simulink model "Simulink_WMM"  (R2021a)
settings: Solver=ode1be  StartTime=0.0  StopTime=350  FixedStep=0.001  RelTol=1e-3
values from neighbouring files (symbols this model uses):
  s = cross(t,r)    [traj_plan_circle.m]
  Y = 0    [traj_plan_3priority.m]    (also in traj_plan_double2.m; traj_plan_ee_8.m; traj_plan_ee_circle.m; traj_plan_scene.m)
undefined symbols (not defined in the file or in its folder): X, Z
libraries: sm_lib x132, nesl_utility x61
(part 1 of 4)
settings Model: PacingRate=0.890000  Creator=zhouz  LastModifiedBy=zhouz

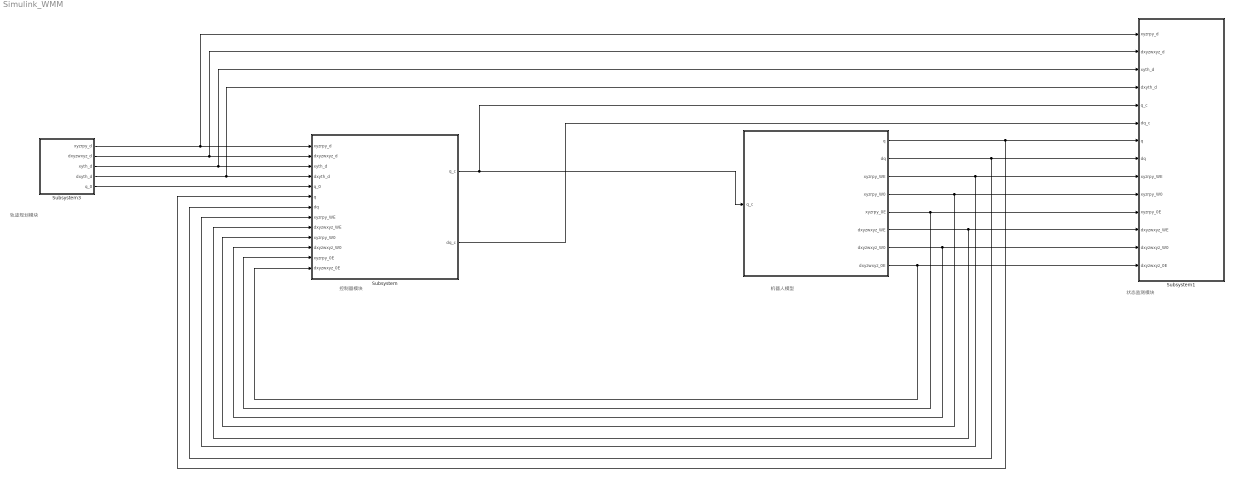
== system Simulink_WMM ==
  note: 机器人模型
  note: 状态监测模块
  note: 控制器模块
  note: 轨迹规划模块
  " " : Subsystem
  Subsystem : Subsystem
  Subsystem1 : Subsystem
  Subsystem3 : Subsystem
  wires:
  Subsystem/2(dq_c) -> Subsystem1/6(dq_c)
  Subsystem3/2(dxyzwxyz_d) -> Subsystem/2(dxyzwxyz_d), Subsystem1/2(dxyzwxyz_d)
  " "/4(xyzrpy_W0) -> Subsystem/10(xyzrpy_W0), Subsystem1/10(xyzrpy_W0)
  Subsystem3/1(xyzrpy_d) -> Subsystem1/1(xyzrpy_d), Subsystem/1(xyzrpy_d)
  Subsystem3/4(dxyth_d) -> Subsystem/4(dxyth_d), Subsystem1/4(dxyth_d)
  Subsystem3/3(xyth_d) -> Subsystem/3(xyth_d), Subsystem1/3(xyth_d)
  " "/8(dxyzwxyz_0E) -> Subsystem1/14(dxyzwxyz_0E), Subsystem/13(dxyzwxyz_0E)
  " "/5(xyzrpy_0E) -> Subsystem/12(xyzrpy_0E), Subsystem1/11(xyzrpy_0E)
  Subsystem/1(q_c) -> " "/1(q_c), Subsystem1/5(q_c)
  " "/7(dxyzwxyz_W0) -> Subsystem1/13(dxyzwxyz_W0), Subsystem/11(dxyzwxyz_W0)
  " "/6(dxyzwxyz_WE) -> Subsystem1/12(dxyzwxyz_WE), Subsystem/9(dxyzwxyz_WE)
  " "/2(dq) -> Subsystem/7(dq), Subsystem1/8(dq)
  " "/1(q) -> Subsystem/6(q), Subsystem1/7(q)
  " "/3(xyzrpy_WE) -> Subsystem/8(xyzrpy_WE), Subsystem1/9(xyzrpy_WE)
  Subsystem3/5(q_0) -> Subsystem/5(q_0)

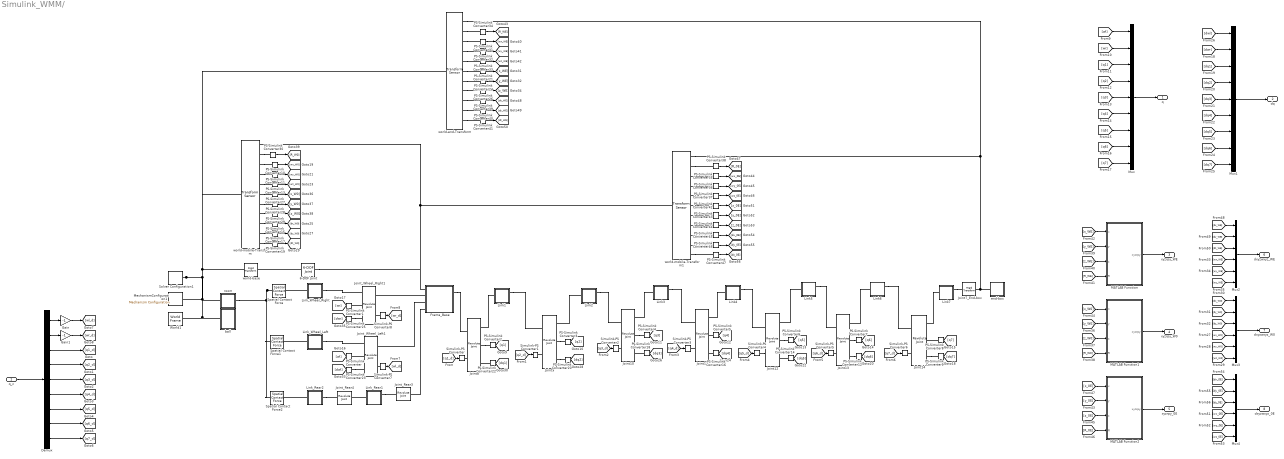
== system Simulink_WMM/  ==
  q_c : Inport
  6-DOF Joint : sm_lib/Joints/6-DOF Joint  JointMode=Normal  SenseConstraintForce=off  SenseConstraintForceX=off  SenseConstraintForceY=off  SenseConstraintForceZ=off  SenseConstraintTorque=off  SenseConstraintTorqueX=off  SenseConstraintTorqueY=off  SenseConstraintTorqueZ=off  SenseTotalForce=off  SenseTotalForceX=off  SenseTotalForceY=off  SenseTotalForceZ=off  SenseTotalTorque=off  SenseTotalTorqueX=off  SenseTotalTorqueY=off  SenseTotalTorqueZ=off  CompositeWrenchDir=FollowerOnBase  CompositeWrenchFrame=BaseFrame  PxEquilibriumPosition=0  PxEquilibriumPositionUnits=m  PxSpringStiffness=0  PxSpringStiffnessUnits=N/m  PxDampingCoefficient=0  PxDampingCoefficientUnits=N/(m/s)  PxTorqueActuationMode=NoTorque  PxMotionActuationMode=ComputedMotion  PxSensePosition=off  PxSenseVelocity=off  PxSenseAcceleration=off  PxSenseTorqueForce=off  PxSenseLowerLimitTorqueForce=off  PxSenseUpperLimitTorqueForce=off  PxLowerLimitSpecify=off  PxLowerLimitBound=-1  PxLowerLimitBoundUnits=m  PxLowerLimitStiffness=1e6  PxLowerLimitStiffnessUnits=N/m  PxLowerLimitDamping=1e3  PxLowerLimitDampingUnits=N/(m/s)  PxLowerLimitTransitionRegionWidth=1e-4  PxLowerLimitTransitionRegionWidthUnits=m  PxUpperLimitSpecify=off  PxUpperLimitBound=1  PxUpperLimitBoundUnits=m  PxUpperLimitStiffness=1e6  PxUpperLimitStiffnessUnits=N/m  PxUpperLimitDamping=1e3  PxUpperLimitDampingUnits=N/(m/s)  PxUpperLimitTransitionRegionWidth=1e-4  PxUpperLimitTransitionRegionWidthUnits=m  PxPositionTargetSpecify=off  PxPositionTargetPriority=High  PxPositionTargetValue=0  PxPositionTargetValueUnits=m  PxVelocityTargetSpecify=off  PxVelocityTargetPriority=High  PxVelocityTargetValue=0  PxVelocityTargetValueUnits=m/s  PyEquilibriumPosition=0  PyEquilibriumPositionUnits=m  PySpringStiffness=0  PySpringStiffnessUnits=N/m  PyDampingCoefficient=0  PyDampingCoefficientUnits=N/(m/s)  PyTorqueActuationMode=NoTorque  PyMotionActuationMode=ComputedMotion  PySensePosition=off  PySenseVelocity=off  PySenseAcceleration=off  PySenseTorqueForce=off  PySenseLowerLimitTorqueForce=off  PySenseUpperLimitTorqueForce=off  PyLowerLimitSpecify=off  PyLowerLimitBound=-1  PyLowerLimitBoundUnits=m  PyLowerLimitStiffness=1e6  PyLowerLimitStiffnessUnits=N/m  PyLowerLimitDamping=1e3  PyLowerLimitDampingUnits=N/(m/s)  PyLowerLimitTransitionRegionWidth=1e-4  PyLowerLimitTransitionRegionWidthUnits=m  PyUpperLimitSpecify=off  PyUpperLimitBound=1  PyUpperLimitBoundUnits=m  PyUpperLimitStiffness=1e6  PyUpperLimitStiffnessUnits=N/m  PyUpperLimitDamping=1e3  PyUpperLimitDampingUnits=N/(m/s)  PyUpperLimitTransitionRegionWidth=1e-4  PyUpperLimitTransitionRegionWidthUnits=m  PyPositionTargetSpecify=off  PyPositionTargetPriority=High  PyPositionTargetValue=0  PyPositionTargetValueUnits=m  PyVelocityTargetSpecify=off  PyVelocityTargetPriority=High  PyVelocityTargetValue=0  PyVelocityTargetValueUnits=m/s  PzEquilibriumPosition=0  PzEquilibriumPositionUnits=m  PzSpringStiffness=0  PzSpringStiffnessUnits=N/m  PzDampingCoefficient=0  PzDampingCoefficientUnits=N/(m/s)  PzTorqueActuationMode=NoTorque  PzMotionActuationMode=ComputedMotion  PzSensePosition=off  PzSenseVelocity=off  PzSenseAcceleration=off  PzSenseTorqueForce=off  PzSenseLowerLimitTorqueForce=off  PzSenseUpperLimitTorqueForce=off  PzLowerLimitSpecify=off  PzLowerLimitBound=-1  PzLowerLimitBoundUnits=m  PzLowerLimitStiffness=1e6  PzLowerLimitStiffnessUnits=N/m  PzLowerLimitDamping=1e3  PzLowerLimitDampingUnits=N/(m/s)  PzLowerLimitTransitionRegionWidth=1e-4  PzLowerLimitTransitionRegionWidthUnits=m  PzUpperLimitSpecify=off  PzUpperLimitBound=1  PzUpperLimitBoundUnits=m  PzUpperLimitStiffness=1e6  PzUpperLimitStiffnessUnits=N/m  PzUpperLimitDamping=1e3  PzUpperLimitDampingUnits=N/(m/s)  PzUpperLimitTransitionRegionWidth=1e-4  PzUpperLimitTransitionRegionWidthUnits=m  PzPositionTargetSpecify=off  PzPositionTargetPriority=High  PzPositionTargetValue=0  PzPositionTargetValueUnits=m  PzVelocityTargetSpecify=off  PzVelocityTargetPriority=High  PzVelocityTargetValue=0  PzVelocityTargetValueUnits=m/s  SphDefPosRotationMethod=None  SphDefPosRotationAngleUnits=deg  SphDefPosRotationStandardAxis=+Z  SphDefPosRotationAngle=0.0  SphDefPosRotationArbitraryAxis=[0 0 1]  SphDefPosFollAlignAxisA=+X  SphDefPosBaseAlignAxisA=+Y  SphDefPosFollAlignAxisB=+Y  SphDefPosBaseAlignAxisB=+Z  SphDefPosRotationSequenceAxes=FollowerAxes  SphDefPosRotationSequence=XYX  SphDefPosRotationSequenceAngles=[0 0 0]  SphDefPosRotationSequenceAnglesUnits=deg  SphDefPosRotationMatrix=[1 0 0; 0 1 0; 0 0 1]  SphEqPosRotationMethod=None  SphEqPosRotationAngleUnits=deg  SphEqPosRotationStandardAxis=+Z  SphEqPosRotationAngle=0.0  SphEqPosRotationArbitraryAxis=[0 0 1]  SphEqPosFollAlignAxisA=+X  SphEqPosBaseAlignAxisA=+Y  SphEqPosFollAlignAxisB=+Y  SphEqPosBaseAlignAxisB=+Z  SphEqPosRotationSequenceAxes=FollowerAxes  SphEqPosRotationSequence=XYX  SphEqPosRotationSequenceAngles=[0 0 0]  SphEqPosRotationSequenceAnglesUnits=deg  SphEqPosRotationMatrix=[1 0 0; 0 1 0; 0 0 1]  SphSpringStiffness=0  SphSpringStiffnessUnits=N*m/deg  SphDampingCoefficient=0  SphDampingCoefficientUnits=N*m/(deg/s)  SphActuateTorqueX=off  SphActuateTorqueY=off  SphActuateTorqueZ=off  SphActuateTorque=off  SphTorqueActuationMode=NoTorque  SphMotionActuationMode=ComputedMotion  SphActuationFrame=BaseFrame  SphSensePosition=off  SphSenseVelocityX=off  SphSenseVelocityY=off  SphSenseVelocityZ=off  SphSenseVelocity=off  SphSenseAccelerationX=off  SphSenseAccelerationY=off  SphSenseAccelerationZ=off  SphSenseAcceleration=off  SphSenseTorqueX=off  SphSenseTorqueY=off  SphSenseTorqueZ=off  SphSenseTorqueForce=off  SphSenseLowerLimitTorqueMag=off  SphSenseUpperLimitTorqueMag=off  SphSensingFrame=BaseFrame  SphLowerLimitSpecify=off  SphLowerLimitBound=15  SphLowerLimitBoundUnits=deg  SphLowerLimitStiffness=1e4  SphLowerLimitStiffnessUnits=N*m/deg  SphLowerLimitDamping=10  SphLowerLimitDampingUnits=N*m/(deg/s)  SphLowerLimitTransitionRegionWidth=0.1  SphLowerLimitTransitionRegionWidthUnits=deg  SphUpperLimitSpecify=off  SphUpperLimitBound=45  SphUpperLimitBoundUnits=deg  SphUpperLimitStiffness=1e4  SphUpperLimitStiffnessUnits=N*m/deg  SphUpperLimitDamping=10  SphUpperLimitDampingUnits=N*m/(deg/s)  SphUpperLimitTransitionRegionWidth=0.1  SphUpperLimitTransitionRegionWidthUnits=deg  SphPositionTargetRotationMethod=None  SphPositionTargetRotationAngleUnits=deg  SphPositionTargetRotationStandardAxis=+Z  SphPositionTargetRotationAngle=0.0  SphPositionTargetRotationArbitraryAxis=[0 0 1]  SphPositionTargetFollAlignAxisA=+X  SphPositionTargetBaseAlignAxisA=+Y  SphPositionTargetFollAlignAxisB=+Y  SphPositionTargetBaseAlignAxisB=+Z  SphPositionTargetRotationSequenceAxes=FollowerAxes  SphPositionTargetRotationSequence=XYX  SphPositionTargetRotationSequenceAngles=[0 0 0]  SphPositionTargetRotationSequenceAnglesUnits=deg  SphPositionTargetRotationMatrix=[1 0 0; 0 1 0; 0 0 1]  SphPositionTargetSpecify=off  SphPositionTargetPriority=High  SphVelocityTargetValue=[0 0 0]  SphVelocityTargetValueUnits=deg/s  SphVelocityTargetSpecify=off  SphVelocityTargetPriority=High  SphVelocityTargetInFollowerFrame=on
  Demux : Demux  Outputs=9
  Frame_Base : Subsystem
  Gain : Gain  Gain=-1
  Gain1 : Gain  Gain=-1
  Joint{8,10,12,14} (4 alike) : sm_lib/Joints/Revolute Joint  JointMode=Normal  SenseConstraintForce=off  SenseConstraintForceX=off  SenseConstraintForceY=off  SenseConstraintForceZ=off  SenseConstraintTorque=off  SenseConstraintTorqueX=off  SenseConstraintTorqueY=off  SenseConstraintTorqueZ=off  SenseTotalForce=off  SenseTotalForceX=off  SenseTotalForceY=off  SenseTotalForceZ=off  SenseTotalTorque=off  SenseTotalTorqueX=off  SenseTotalTorqueY=off  SenseTotalTorqueZ=off  CompositeWrenchDir=FollowerOnBase  CompositeWrenchFrame=BaseFrame  EquilibriumPosition=0  EquilibriumPositionUnits=deg  SpringStiffness=0  SpringStiffnessUnits=N*m/deg  DampingCoefficient=0  DampingCoefficientUnits=m^2*kg/s/rad  TorqueActuationMode=ComputedTorque  MotionActuationMode=InputMotion  SensePosition=on  SenseVelocity=on  SenseAcceleration=off  SenseTorqueForce=off  SenseLowerLimitTorqueForce=off  SenseUpperLimitTorqueForce=off  LowerLimitSpecify=off  LowerLimitBound=0  LowerLimitBoundUnits=rad  LowerLimitStiffness=1e4  LowerLimitStiffnessUnits=N*m/deg  LowerLimitDamping=10  LowerLimitDampingUnits=N*m/(deg/s)  LowerLimitTransitionRegionWidth=0.1  LowerLimitTransitionRegionWidthUnits=deg  UpperLimitSpecify=off  UpperLimitBound=0  UpperLimitBoundUnits=rad  UpperLimitStiffness=1e4  UpperLimitStiffnessUnits=N*m/deg  UpperLimitDamping=10  UpperLimitDampingUnits=N*m/(deg/s)  UpperLimitTransitionRegionWidth=0.1  UpperLimitTransitionRegionWidthUnits=deg  PositionTargetSpecify=on  PositionTargetPriority=Low  PositionTargetValue=0  PositionTargetValueUnits=rad  VelocityTargetSpecify=on  VelocityTargetPriority=Low  VelocityTargetValue=0  VelocityTargetValueUnits=rad/s
  Joint11 : sm_lib/Joints/Revolute Joint  JointMode=Normal  SenseConstraintForce=off  SenseConstraintForceX=off  SenseConstraintForceY=off  SenseConstraintForceZ=off  SenseConstraintTorque=off  SenseConstraintTorqueX=off  SenseConstraintTorqueY=off  SenseConstraintTorqueZ=off  SenseTotalForce=off  SenseTotalForceX=off  SenseTotalForceY=off  SenseTotalForceZ=off  SenseTotalTorque=off  SenseTotalTorqueX=off  SenseTotalTorqueY=off  SenseTotalTorqueZ=off  CompositeWrenchDir=FollowerOnBase  CompositeWrenchFrame=BaseFrame  EquilibriumPosition=0  EquilibriumPositionUnits=deg  SpringStiffness=0  SpringStiffnessUnits=N*m/deg  DampingCoefficient=0  DampingCoefficientUnits=m^2*kg/s/rad  TorqueActuationMode=ComputedTorque  MotionActuationMode=InputMotion  SensePosition=on  SenseVelocity=on  SenseAcceleration=off  SenseTorqueForce=off  SenseLowerLimitTorqueForce=off  SenseUpperLimitTorqueForce=off  LowerLimitSpecify=on  LowerLimitBound=-147  LowerLimitBoundUnits=deg  LowerLimitStiffness=1e4  LowerLimitStiffnessUnits=N*m/deg  LowerLimitDamping=10  LowerLimitDampingUnits=N*m/(deg/s)  LowerLimitTransitionRegionWidth=0.1  LowerLimitTransitionRegionWidthUnits=deg  UpperLimitSpecify=on  UpperLimitBound=147  UpperLimitBoundUnits=rad  UpperLimitStiffness=1e4  UpperLimitStiffnessUnits=N*m/deg  UpperLimitDamping=10  UpperLimitDampingUnits=N*m/(deg/s)  UpperLimitTransitionRegionWidth=0.1  UpperLimitTransitionRegionWidthUnits=deg  PositionTargetSpecify=on  PositionTargetPriority=Low  PositionTargetValue=0  PositionTargetValueUnits=rad  VelocityTargetSpecify=on  VelocityTargetPriority=Low  VelocityTargetValue=0  VelocityTargetValueUnits=rad/s
  Joint13 : sm_lib/Joints/Revolute Joint  JointMode=Normal  SenseConstraintForce=off  SenseConstraintForceX=off  SenseConstraintForceY=off  SenseConstraintForceZ=off  SenseConstraintTorque=off  SenseConstraintTorqueX=off  SenseConstraintTorqueY=off  SenseConstraintTorqueZ=off  SenseTotalForce=off  SenseTotalForceX=off  SenseTotalForceY=off  SenseTotalForceZ=off  SenseTotalTorque=off  SenseTotalTorqueX=off  SenseTotalTorqueY=off  SenseTotalTorqueZ=off  CompositeWrenchDir=FollowerOnBase  CompositeWrenchFrame=BaseFrame  EquilibriumPosition=0  EquilibriumPositionUnits=deg  SpringStiffness=0  SpringStiffnessUnits=N*m/deg  DampingCoefficient=0  DampingCoefficientUnits=m^2*kg/s/rad  TorqueActuationMode=ComputedTorque  MotionActuationMode=InputMotion  SensePosition=on  SenseVelocity=on  SenseAcceleration=off  SenseTorqueForce=off  SenseLowerLimitTorqueForce=off  SenseUpperLimitTorqueForce=off  LowerLimitSpecify=on  LowerLimitBound=-117  LowerLimitBoundUnits=rad  LowerLimitStiffness=1e4  LowerLimitStiffnessUnits=N*m/deg  LowerLimitDamping=10  LowerLimitDampingUnits=N*m/(deg/s)  LowerLimitTransitionRegionWidth=0.1  LowerLimitTransitionRegionWidthUnits=deg  UpperLimitSpecify=on  UpperLimitBound=117  UpperLimitBoundUnits=rad  UpperLimitStiffness=1e4  UpperLimitStiffnessUnits=N*m/deg  UpperLimitDamping=10  UpperLimitDampingUnits=N*m/(deg/s)  UpperLimitTransitionRegionWidth=0.1  UpperLimitTransitionRegionWidthUnits=deg  PositionTargetSpecify=on  PositionTargetPriority=Low  PositionTargetValue=0  PositionTargetValueUnits=rad  VelocityTargetSpecify=on  VelocityTargetPriority=Low  VelocityTargetValue=0  VelocityTargetValueUnits=rad/s
  Joint7_End-box : sm_lib/Frames and Transforms/Rigid Transform  TranslationMethod=Cartesian  TranslationStandardOffset=0  TranslationLengthUnit=m  TranslationStandardAxis=+Z  TranslationCartesianOffset=[0, 0, 0.2374]  TranslationROffset=0  TranslationROffsetUnits=m  TranslationZOffset=0  TranslationZOffsetUnits=m  TranslationThetaOffset=0  TranslationThetaOffsetUnits=deg  RotationMethod=ArbitraryAxis  RotationAngleUnits=rad  RotationStandardAxis=+Z  RotationAngle=0  RotationArbitraryAxis=[1, 0, 0]  FollAlignAxisA=+X  BaseAlignAxisA=+Y  FollAlignAxisB=+Y  BaseAlignAxisB=+Z  RotationSequenceAxes=FollowerAxes  RotationSequence=XYX  RotationSequenceAngles=[0 0 0]  RotationSequenceAnglesUnits=deg  RotationMatrix=[1 0 0; 0 1 0; 0 0 1]
  Joint9 : sm_lib/Joints/Revolute Joint  JointMode=Normal  SenseConstraintForce=off  SenseConstraintForceX=off  SenseConstraintForceY=off  SenseConstraintForceZ=off  SenseConstraintTorque=off  SenseConstraintTorqueX=off  SenseConstraintTorqueY=off  SenseConstraintTorqueZ=off  SenseTotalForce=off  SenseTotalForceX=off  SenseTotalForceY=off  SenseTotalForceZ=off  SenseTotalTorque=off  SenseTotalTorqueX=off  SenseTotalTorqueY=off  SenseTotalTorqueZ=off  CompositeWrenchDir=FollowerOnBase  CompositeWrenchFrame=BaseFrame  EquilibriumPosition=0  EquilibriumPositionUnits=deg  SpringStiffness=0  SpringStiffnessUnits=N*m/deg  DampingCoefficient=0  DampingCoefficientUnits=m^2*kg/s/rad  TorqueActuationMode=ComputedTorque  MotionActuationMode=InputMotion  SensePosition=on  SenseVelocity=on  SenseAcceleration=off  SenseTorqueForce=off  SenseLowerLimitTorqueForce=off  SenseUpperLimitTorqueForce=off  LowerLimitSpecify=on  LowerLimitBound=-126  LowerLimitBoundUnits=deg  LowerLimitStiffness=1e4  LowerLimitStiffnessUnits=N*m/deg  LowerLimitDamping=10  LowerLimitDampingUnits=N*m/(deg/s)  LowerLimitTransitionRegionWidth=0.1  LowerLimitTransitionRegionWidthUnits=deg  UpperLimitSpecify=on  UpperLimitBound=126  UpperLimitBoundUnits=deg  UpperLimitStiffness=1e4  UpperLimitStiffnessUnits=N*m/deg  UpperLimitDamping=10  UpperLimitDampingUnits=N*m/(deg/s)  UpperLimitTransitionRegionWidth=0.1  UpperLimitTransitionRegionWidthUnits=deg  PositionTargetSpecify=on  PositionTargetPriority=Low  PositionTargetValue=0  PositionTargetValueUnits=rad  VelocityTargetSpecify=on  VelocityTargetPriority=Low  VelocityTargetValue=0  VelocityTargetValueUnits=rad/s
  Joint_Rear3 : sm_lib/Joints/Revolute Joint  JointMode=Normal  SenseConstraintForce=off  SenseConstraintForceX=off  SenseConstraintForceY=off  SenseConstraintForceZ=off  SenseConstraintTorque=off  SenseConstraintTorqueX=off  SenseConstraintTorqueY=off  SenseConstraintTorqueZ=off  SenseTotalForce=off  SenseTotalForceX=off  SenseTotalForceY=off  SenseTotalForceZ=off  SenseTotalTorque=off  SenseTotalTorqueX=off  SenseTotalTorqueY=off  SenseTotalTorqueZ=off  CompositeWrenchDir=FollowerOnBase  CompositeWrenchFrame=BaseFrame  EquilibriumPosition=0  EquilibriumPositionUnits=deg  SpringStiffness=0  SpringStiffnessUnits=N*m/deg  DampingCoefficient=2  DampingCoefficientUnits=N*m/(deg/s)  TorqueActuationMode=NoTorque  MotionActuationMode=ComputedMotion  SensePosition=off  SenseVelocity=off  SenseAcceleration=off  SenseTorqueForce=off  SenseLowerLimitTorqueForce=off  SenseUpperLimitTorqueForce=off  LowerLimitSpecify=off  LowerLimitBound=0  LowerLimitBoundUnits=rad  LowerLimitStiffness=1e4  LowerLimitStiffnessUnits=N*m/deg  LowerLimitDamping=10  LowerLimitDampingUnits=N*m/(deg/s)  LowerLimitTransitionRegionWidth=0.1  LowerLimitTransitionRegionWidthUnits=deg  UpperLimitSpecify=off  UpperLimitBound=0  UpperLimitBoundUnits=rad  UpperLimitStiffness=1e4  UpperLimitStiffnessUnits=N*m/deg  UpperLimitDamping=10  UpperLimitDampingUnits=N*m/(deg/s)  UpperLimitTransitionRegionWidth=0.1  UpperLimitTransitionRegionWidthUnits=deg  PositionTargetSpecify=on  PositionTargetPriority=Low  PositionTargetValue=0  PositionTargetValueUnits=rad  VelocityTargetSpecify=on  VelocityTargetPriority=Low  VelocityTargetValue=0  VelocityTargetValueUnits=rad/s
  Joint_Rear4 : sm_lib/Joints/Revolute Joint  JointMode=Normal  SenseConstraintForce=off  SenseConstraintForceX=off  SenseConstraintForceY=off  SenseConstraintForceZ=off  SenseConstraintTorque=off  SenseConstraintTorqueX=off  SenseConstraintTorqueY=off  SenseConstraintTorqueZ=off  SenseTotalForce=off  SenseTotalForceX=off  SenseTotalForceY=off  SenseTotalForceZ=off  SenseTotalTorque=off  SenseTotalTorqueX=off  SenseTotalTorqueY=off  SenseTotalTorqueZ=off  CompositeWrenchDir=FollowerOnBase  CompositeWrenchFrame=BaseFrame  EquilibriumPosition=0  EquilibriumPositionUnits=deg  SpringStiffness=0  SpringStiffnessUnits=N*m/deg  DampingCoefficient=0  DampingCoefficientUnits=N*m/(deg/s)  TorqueActuationMode=NoTorque  MotionActuationMode=ComputedMotion  SensePosition=off  SenseVelocity=off  SenseAcceleration=off  SenseTorqueForce=off  SenseLowerLimitTorqueForce=off  SenseUpperLimitTorqueForce=off  LowerLimitSpecify=off  LowerLimitBound=0  LowerLimitBoundUnits=rad  LowerLimitStiffness=1e4  LowerLimitStiffnessUnits=N*m/deg  LowerLimitDamping=10  LowerLimitDampingUnits=N*m/(deg/s)  LowerLimitTransitionRegionWidth=0.1  LowerLimitTransitionRegionWidthUnits=deg  UpperLimitSpecify=off  UpperLimitBound=0  UpperLimitBoundUnits=rad  UpperLimitStiffness=1e4  UpperLimitStiffnessUnits=N*m/deg  UpperLimitDamping=10  UpperLimitDampingUnits=N*m/(deg/s)  UpperLimitTransitionRegionWidth=0.1  UpperLimitTransitionRegionWidthUnits=deg  PositionTargetSpecify=on  PositionTargetPriority=Low  PositionTargetValue=0  PositionTargetValueUnits=rad  VelocityTargetSpecify=on  VelocityTargetPriority=Low  VelocityTargetValue=0  VelocityTargetValueUnits=rad/s
  Joint_Wheel_Left1 : sm_lib/Joints/Revolute Joint  JointMode=Normal  SenseConstraintForce=off  SenseConstraintForceX=off  SenseConstraintForceY=off  SenseConstraintForceZ=off  SenseConstraintTorque=off  SenseConstraintTorqueX=off  SenseConstraintTorqueY=off  SenseConstraintTorqueZ=off  SenseTotalForce=off  SenseTotalForceX=off  SenseTotalForceY=off  SenseTotalForceZ=off  SenseTotalTorque=off  SenseTotalTorqueX=off  SenseTotalTorqueY=off  SenseTotalTorqueZ=off  CompositeWrenchDir=FollowerOnBase  CompositeWrenchFrame=BaseFrame  EquilibriumPosition=0  EquilibriumPositionUnits=deg  SpringStiffness=0  SpringStiffnessUnits=N*m/deg  DampingCoefficient=0  DampingCoefficientUnits=N*m/(deg/s)  TorqueActuationMode=ComputedTorque  MotionActuationMode=InputMotion  SensePosition=on  SenseVelocity=on  SenseAcceleration=off  SenseTorqueForce=off  SenseLowerLimitTorqueForce=off  SenseUpperLimitTorqueForce=off  LowerLimitSpecify=off  LowerLimitBound=0  LowerLimitBoundUnits=rad  LowerLimitStiffness=1e4  LowerLimitStiffnessUnits=N*m/deg  LowerLimitDamping=10  LowerLimitDampingUnits=N*m/(deg/s)  LowerLimitTransitionRegionWidth=0.1  LowerLimitTransitionRegionWidthUnits=deg  UpperLimitSpecify=off  UpperLimitBound=0  UpperLimitBoundUnits=rad  UpperLimitStiffness=1e4  UpperLimitStiffnessUnits=N*m/deg  UpperLimitDamping=10  UpperLimitDampingUnits=N*m/(deg/s)  UpperLimitTransitionRegionWidth=0.1  UpperLimitTransitionRegionWidthUnits=deg  PositionTargetSpecify=on  PositionTargetPriority=Low  PositionTargetValue=0  PositionTargetValueUnits=rad  VelocityTargetSpecify=on  VelocityTargetPriority=Low  VelocityTargetValue=0  VelocityTargetValueUnits=rad/s
  Joint_Wheel_Right1 : sm_lib/Joints/Revolute Joint  JointMode=Normal  SenseConstraintForce=off  SenseConstraintForceX=off  SenseConstraintForceY=off  SenseConstraintForceZ=off  SenseConstraintTorque=off  SenseConstraintTorqueX=off  SenseConstraintTorqueY=off  SenseConstraintTorqueZ=off  SenseTotalForce=off  SenseTotalForceX=off  SenseTotalForceY=off  SenseTotalForceZ=off  SenseTotalTorque=off  SenseTotalTorqueX=off  SenseTotalTorqueY=off  SenseTotalTorqueZ=off  CompositeWrenchDir=FollowerOnBase  CompositeWrenchFrame=BaseFrame  EquilibriumPosition=0  EquilibriumPositionUnits=deg  SpringStiffness=0  SpringStiffnessUnits=N*m/deg  DampingCoefficient=0  DampingCoefficientUnits=N*m/(deg/s)  TorqueActuationMode=ComputedTorque  MotionActuationMode=InputMotion  SensePosition=on  SenseVelocity=on  SenseAcceleration=off  SenseTorqueForce=off  SenseLowerLimitTorqueForce=off  SenseUpperLimitTorqueForce=off  LowerLimitSpecify=off  LowerLimitBound=0  LowerLimitBoundUnits=rad  LowerLimitStiffness=1e4  LowerLimitStiffnessUnits=N*m/deg  LowerLimitDamping=10  LowerLimitDampingUnits=N*m/(deg/s)  LowerLimitTransitionRegionWidth=0.1  LowerLimitTransitionRegionWidthUnits=deg  UpperLimitSpecify=off  UpperLimitBound=0  UpperLimitBoundUnits=rad  UpperLimitStiffness=1e4  UpperLimitStiffnessUnits=N*m/deg  UpperLimitDamping=10  UpperLimitDampingUnits=N*m/(deg/s)  UpperLimitTransitionRegionWidth=0.1  UpperLimitTransitionRegionWidthUnits=deg  PositionTargetSpecify=on  PositionTargetPriority=Low  PositionTargetValue=0  PositionTargetValueUnits=rad  VelocityTargetSpecify=on  VelocityTargetPriority=Low  VelocityTargetValue=0  VelocityTargetValueUnits=rad/s
  Link1 : Subsystem
  Link2 : Subsystem
  Link3 : Subsystem
  Link4 : Subsystem
  Link5 : Subsystem
  Link6 : Subsystem
  Link7 : Subsystem
  Link_Rear1 : Subsystem
  Link_Rear2 : Subsystem
  Link_Wheel_Left : Subsystem
  Link_Wheel_Right : Subsystem
  MATLAB Function : MATLAB Function  TreatAsAtomicUnit=on
  MATLAB Function1 : MATLAB Function  TreatAsAtomicUnit=on
  MATLAB Function2 : MATLAB Function  TreatAsAtomicUnit=on
  MechanismConfiguration1 : sm_lib/Utilities/Mechanism Configuration  UniformGravity=Constant  GravityVector=[0 0 -9.80665]  GravityVectorUnits=m/s^2  GravityUnits=m/s^2  LinearizationDelta=0.001  JointModeTransitionNonlinearIterations=2
  Mux : Mux  Inputs=9
  Mux1 : Mux  Inputs=9
  Mux2 : Mux  Inputs=6
  Mux3 : Mux  Inputs=6
  Mux4 : Mux  Inputs=6
  PS-Simulink Converter{,1..47} (48 alike) : nesl_utility/PS-Simulink Converter  PhysicalDomain=network_engine_domain  SubClassName=ps_output  LeftPortType=input  RightPortType=output  PseudoPeriodic=off  Frequencies=[]  Unit=inherit  AffineConversion=off
      settings: SourceProductBaseCode=PW,SS
  Simulink-PS Converter{,1..8} (9 alike) : nesl_utility/Simulink-PS Converter  PhysicalDomain=network_engine_domain  SubClassName=ps_input  LeftPortType=input  RightPortType=output  PseudoPeriodic=off  Frequencies=[]  NoiseDistribution=none  NoiseParameters=[]  Unit=rad  AffineConversion=off  FilteringAndDerivatives=filter  SimscapeFilterOrder=2  InputFilterTimeConstant=0.001  UdotUserProvided=0
      settings: SourceProductBaseCode=PW,SS
  Solver Configuration1 : nesl_utility/Solver Configuration  PhysicalDomain=network_engine_domain  SubClassName=solver  LeftPortType=input  RightPortType=generic  Tones=[]  Harmonics=[]  SimulateNoise=off  Profile=off  UseLocalSampling=off  EnableSwitchedLinearOptims=on  FrequencyDomain=off  UseCCode=off  RelTol=0.001  AbsTol=1e-06  MinStep=1e-09  ToWorkspace=off  RevertToSquareIcSolve=off  NumHomotopyIterations=100  PhasorMode=off  PhasorModeNumHarmonics=1  DoDC=off  ResidualTolerance=1e-09  UseLocalSolver=off  LocalSolverChoice=NE_BACKWARD_EULER_ADVANCER  LocalSolverSampleTime=0.001  DoFixedCost=off  MaxNonlinIter=3  MaxModeIter=2  ComputeImpulses=off  ImpulseIterations=2  LinearAlgebra=auto  EquationFormulation=NE_TIME_EF  DelaysMemoryBudget=1024  AutomaticFiltering=on  FilteringTimeConstant=0.001  PartitionStorageMethod=AS_NEEDED  PartitionMemoryBudget=1024  PartitionMethod=ROBUST
      settings: SourceProductBaseCode=PW,SS
  Spatial Contact Force : sm_lib/Forces and Torques/Spatial Contact Force  CoefficientOfDynamicFriction=0.3  CoefficientOfStaticFriction=0.5  SenseContactBaseRotation=off  SenseContactBaseTranslation=off  NormalDamping=1e3  NormalDampingUnits=N/(m/s)  SenseContactFollowerRotation=off  SenseContactFollowerTranslation=off  SenseContactSignal=off  NormalStiffness=1e6  NormalStiffnessUnits=N/m  FrictionalCriticalVelocity=1e-3  FrictionalCriticalVelocityUnits=m/s  ZeroCrossDetectContactStartAndEnd=off  FrictionType=SmoothStickSlip  SenseFrictionalForceMagnitude=off  SenseNormalForceMagnitude=off  NormalForceType=SmoothSpringDamper  SenseNormalVelocity=off  SenseSeparationDistance=off  SenseTangentialVelocity=off  SenseTangentialVelocityMagnitude=off  NormalTransitionRegionWidth=1e-4  NormalTransitionRegionWidthUnits=m
  Spatial Contact Force1 : sm_lib/Forces and Torques/Spatial Contact Force  CoefficientOfDynamicFriction=0.3  CoefficientOfStaticFriction=0.5  SenseContactBaseRotation=off  SenseContactBaseTranslation=off  NormalDamping=1e3  NormalDampingUnits=N/(m/s)  SenseContactFollowerRotation=off  SenseContactFollowerTranslation=off  SenseContactSignal=off  NormalStiffness=1e6  NormalStiffnessUnits=N/m  FrictionalCriticalVelocity=1e-3  FrictionalCriticalVelocityUnits=m/s  ZeroCrossDetectContactStartAndEnd=off  FrictionType=SmoothStickSlip  SenseFrictionalForceMagnitude=off  SenseNormalForceMagnitude=off  NormalForceType=SmoothSpringDamper  SenseNormalVelocity=off  SenseSeparationDistance=off  SenseTangentialVelocity=off  SenseTangentialVelocityMagnitude=off  NormalTransitionRegionWidth=1e-4  NormalTransitionRegionWidthUnits=m
  Spatial Contact Force2 : sm_lib/Forces and Torques/Spatial Contact Force  CoefficientOfDynamicFriction=0.3  CoefficientOfStaticFriction=0.5  SenseContactBaseRotation=off  SenseContactBaseTranslation=off  NormalDamping=1e3  NormalDampingUnits=N/(m/s)  SenseContactFollowerRotation=off  SenseContactFollowerTranslation=off  SenseContactSignal=off  NormalStiffness=1e6  NormalStiffnessUnits=N/m  FrictionalCriticalVelocity=1e-3  FrictionalCriticalVelocityUnits=m/s  ZeroCrossDetectContactStartAndEnd=off  FrictionType=SmoothStickSlip  SenseFrictionalForceMagnitude=off  SenseNormalForceMagnitude=off  NormalForceType=SmoothSpringDamper  SenseNormalVelocity=off  SenseSeparationDistance=off  SenseTangentialVelocity=off  SenseTangentialVelocityMagnitude=off  NormalTransitionRegionWidth=1e-4  NormalTransitionRegionWidthUnits=m
  World1 : sm_lib/Frames and Transforms/World Frame
  ball : Subsystem
  end-box : Subsystem
  room : Subsystem
  world-base : sm_lib/Frames and Transforms/Rigid Transform  TranslationMethod=Cartesian  TranslationStandardOffset=0  TranslationLengthUnit=m  TranslationStandardAxis=+Z  TranslationCartesianOffset=[0 0 0.4]  TranslationROffset=0  TranslationROffsetUnits=m  TranslationZOffset=0  TranslationZOffsetUnits=m  TranslationThetaOffset=0  TranslationThetaOffsetUnits=deg  RotationMethod=None  RotationAngleUnits=deg  RotationStandardAxis=+Z  RotationAngle=0.0  RotationArbitraryAxis=[0 0 1]  FollAlignAxisA=+X  BaseAlignAxisA=+Y  FollAlignAxisB=+Y  BaseAlignAxisB=+Z  RotationSequenceAxes=FollowerAxes  RotationSequence=XYX  RotationSequenceAngles=[0 0 0]  RotationSequenceAnglesUnits=deg  RotationMatrix=[1 0 0; 0 1 0; 0 0 1]
  world-end-Transform : sm_lib/Frames and Transforms/Transform Sensor  MeasurementFrame=World  SenseAngle=off  SenseAxis=off  SenseAngle1=off  SenseAngle2=off  SenseAngle3=off  SenseQ=off  SenseR=on  SenseOmegaX=on  SenseOmegaY=on  SenseOmegaZ=on  SenseOmega1=off  SenseOmega2=off  SenseOmega3=off  SenseQDot=off  SenseRDot=off  SenseAlphaX=off  SenseAlphaY=off  SenseAlphaZ=off  SenseAlpha1=off  SenseAlpha2=off  SenseAlpha3=off  SenseQDDot=off  SenseRDDot=off  SenseX=on  SenseY=on  SenseZ=on  SenseRad=off  SenseAzim=off  SenseDist=off  SenseInc=off  SenseXDot=on  SenseYDot=on  SenseZDot=on  SenseRadDot=off  SenseAzimDot=off  SenseDistDot=off  SenseIncDot=off  SenseXDDot=off  SenseYDDot=off  SenseZDDot=off  SenseRadDDot=off  SenseAzimDDot=off  SenseDistDDot=off  SenseIncDDot=off
  world-mobile-Transform : sm_lib/Frames and Transforms/Transform Sensor  MeasurementFrame=World  SenseAngle=off  SenseAxis=off  SenseAngle1=off  SenseAngle2=off  SenseAngle3=off  SenseQ=off  SenseR=on  SenseOmegaX=on  SenseOmegaY=on  SenseOmegaZ=on  SenseOmega1=off  SenseOmega2=off  SenseOmega3=off  SenseQDot=off  SenseRDot=off  SenseAlphaX=off  SenseAlphaY=off  SenseAlphaZ=off  SenseAlpha1=off  SenseAlpha2=off  SenseAlpha3=off  SenseQDDot=off  SenseRDDot=off  SenseX=on  SenseY=on  SenseZ=on  SenseRad=off  SenseAzim=off  SenseDist=off  SenseInc=off  SenseXDot=on  SenseYDot=on  SenseZDot=on  SenseRadDot=off  SenseAzimDot=off  SenseDistDot=off  SenseIncDot=off  SenseXDDot=off  SenseYDDot=off  SenseZDDot=off  SenseRadDDot=off  SenseAzimDDot=off  SenseDistDDot=off  SenseIncDDot=off
  world-mobile-Transform1 : sm_lib/Frames and Transforms/Transform Sensor  MeasurementFrame=Base  SenseAngle=off  SenseAxis=off  SenseAngle1=off  SenseAngle2=off  SenseAngle3=off  SenseQ=off  SenseR=on  SenseOmegaX=on  SenseOmegaY=on  SenseOmegaZ=on  SenseOmega1=off  SenseOmega2=off  SenseOmega3=off  SenseQDot=off  SenseRDot=off  SenseAlphaX=off  SenseAlphaY=off  SenseAlphaZ=off  SenseAlpha1=off  SenseAlpha2=off  SenseAlpha3=off  SenseQDDot=off  SenseRDDot=off  SenseX=on  SenseY=on  SenseZ=on  SenseRad=off  SenseAzim=off  SenseDist=off  SenseInc=off  SenseXDot=on  SenseYDot=on  SenseZDot=on  SenseRadDot=off  SenseAzimDot=off  SenseDistDot=off  SenseIncDot=off  SenseXDDot=off  SenseYDDot=off  SenseZDDot=off  SenseRadDDot=off  SenseAzimDDot=off  SenseDistDDot=off  SenseIncDDot=off
  q : Outport
  dq : Outport  Port=2
  xyzrpy_WE : Outport  Port=3
  xyzrpy_W0 : Outport  Port=4
  xyzrpy_0E : Outport  Port=5
  dxyzwxyz_WE : Outport  Port=6
  dxyzwxyz_W0 : Outport  Port=7
  dxyzwxyz_0E : Outport  Port=8
  wires:
  PS-Simulink Converter32/1 -> [wy_WE]
  PS-Simulink Converter4/1 -> [q3]
  [q4] -> Mux/6
  Demux/9 -> [q7_d]
  Mux/1 -> q/1
  q_c/1 -> Demux/1
  PS-Simulink Converter33/1 -> [wz_WE]
  PS-Simulink Converter14/1 -> [dq5]
  Demux/7 -> [q5_d]
  Demux/6 -> [q4_d]
  [dq4] -> Mux1/6
  Demux/8 -> [q6_d]
  PS-Simulink Converter22/1 -> [dq1]
  PS-Simulink Converter34/1 -> [R_WE]
  PS-Simulink Converter3/1 -> [q2]
  [dwl] -> Mux1/1
  Demux/4 -> [q2_d]
  PS-Simulink Converter12/1 -> [dq6]
  [dq6] -> Mux1/8
  PS-Simulink Converter28/1 -> [y_W0]
  PS-Simulink Converter25/1 -> [dwr]
  PS-Simulink Converter9/1 -> [dq7]
  [q1] -> Mux/3
  [dq1] -> Mux1/3
  [dq7] -> Mux1/9
  PS-Simulink Converter38/1 -> [R_0E]
  PS-Simulink Converter27/1 -> [x_W0]
  PS-Simulink Converter29/1 -> [z_W0]
  [q7_d] -> Simulink-PS Converter6/1
  PS-Simulink Converter36/1 -> [wy_0E]
  PS-Simulink Converter37/1 -> [wz_0E]
  [q2_d] -> Simulink-PS Converter1/1
  [q7] -> Mux/9
  PS-Simulink Converter5/1 -> [q4]
  PS-Simulink Converter20/1 -> [dq2]
  PS-Simulink Converter30/1 -> [R_W0]
  [q6_d] -> Simulink-PS Converter5/1
  PS-Simulink Converter18/1 -> [dq3]
  PS-Simulink Converter35/1 -> [wx_0E]
  [wl_d] -> Simulink-PS Converter7/1
  PS-Simulink Converter8/1 -> [q7]
  PS-Simulink Converter7/1 -> [q6]
  Demux/1 -> Gain/1
  [dq5] -> Mux1/7
  [dq2] -> Mux1/4
  [wl] -> Mux/1
  PS-Simulink Converter2/1 -> [q1]
  [q5] -> Mux/7
  PS-Simulink Converter/1 -> [wl]
  [q5_d] -> Simulink-PS Converter4/1
  PS-Simulink Converter1/1 -> [wr]
  [q6] -> Mux/8
  [q4_d] -> Simulink-PS Converter3/1
  [q2] -> Mux/4
  [dwr] -> Mux1/2
  Demux/3 -> [q1_d]
  Demux/2 -> Gain1/1
  [wr_d] -> Simulink-PS Converter8/1
  PS-Simulink Converter31/1 -> [wx_WE]
  [q3] -> Mux/5
  [wr] -> Mux/2
  [q3_d] -> Simulink-PS Converter2/1
  PS-Simulink Converter23/1 -> [dwl]
  PS-Simulink Converter6/1 -> [q5]
  PS-Simulink Converter16/1 -> [dq4]
  [q1_d] -> Simulink-PS Converter/1
  [dq3] -> Mux1/5
  Demux/5 -> [q3_d]
  Gain/1 -> [wl_d]
  Gain1/1 -> [wr_d]
  Mux1/1 -> dq/1
  MATLAB Function/1(xyzrpy) -> xyzrpy_WE/1
  [z_WE] -> MATLAB Function/3(z)
  [x_WE] -> MATLAB Function/1(x)
  [y_WE] -> MATLAB Function/2(y)
  [R_WE] -> MATLAB Function/4(R)
  [R_W0] -> MATLAB Function1/4(R)
  [y_W0] -> MATLAB Function1/2(y)
  [x_W0] -> MATLAB Function1/1(x)
  [z_W0] -> MATLAB Function1/3(z)
  MATLAB Function1/1(xyzrpy) -> xyzrpy_W0/1
  [R_0E] -> MATLAB Function2/4(R)
  [x_0E] -> MATLAB Function2/1(x)
  [y_0E] -> MATLAB Function2/2(y)
  [z_0E] -> MATLAB Function2/3(z)
  MATLAB Function2/1(xyzrpy) -> xyzrpy_0E/1
  PS-Simulink Converter13/1 -> [wz_W0]
  PS-Simulink Converter10/1 -> [wx_W0]
  PS-Simulink Converter11/1 -> [wy_W0]
  PS-Simulink Converter19/1 -> [dz_W0]
  PS-Simulink Converter15/1 -> [dx_W0]
  PS-Simulink Converter17/1 -> [dy_W0]
  PS-Simulink Converter21/1 -> [x_WE]
  PS-Simulink Converter26/1 -> [z_WE]
  PS-Simulink Converter24/1 -> [y_WE]
  PS-Simulink Converter40/1 -> [dy_WE]
  PS-Simulink Converter41/1 -> [dz_WE]
  PS-Simulink Converter39/1 -> [dx_WE]
  PS-Simulink Converter42/1 -> [x_0E]
  PS-Simulink Converter44/1 -> [z_0E]
  PS-Simulink Converter43/1 -> [y_0E]
  PS-Simulink Converter46/1 -> [dy_0E]
  PS-Simulink Converter47/1 -> [dz_0E]
  PS-Simulink Converter45/1 -> [dx_0E]
  [dx_WE] -> Mux2/1
  [dy_WE] -> Mux2/2
  [dz_WE] -> Mux2/3
  [wx_WE] -> Mux2/4
  [wy_WE] -> Mux2/5
  [wz_WE] -> Mux2/6
  Mux2/1 -> dxyzwxyz_WE/1
  Mux3/1 -> dxyzwxyz_W0/1
  [wz_W0] -> Mux3/6
  [wy_W0] -> Mux3/5
  [wx_W0] -> Mux3/4
  [dz_W0] -> Mux3/3
  [dy_W0] -> Mux3/2
  [dx_W0] -> Mux3/1
  [dx_0E] -> Mux4/1
  [dy_0E] -> Mux4/2
  [dz_0E] -> Mux4/3
  [wx_0E] -> Mux4/4
  [wy_0E] -> Mux4/5
  [wz_0E] -> Mux4/6
  Mux4/1 -> dxyzwxyz_0E/1
  connections:
  Joint13/RConn2 -- PS-Simulink Converter7/LConn1
  Frame_Base/LConn2 -- Joint_Wheel_Right1/LConn1
  world-end-Transform/RConn3 -- PS-Simulink Converter31/LConn1
  PS-Simulink Converter8/LConn1 -- Joint14/RConn2
  Simulink-PS Converter5/RConn1 -- Joint13/LConn2
  Link_Rear1/LConn1 -- Joint_Rear3/RConn1
  world-end-Transform/RConn4 -- PS-Simulink Converter32/LConn1
  Link4/LConn1 -- Joint11/RConn1
  world-end-Transform/RConn2 -- PS-Simulink Converter34/LConn1
  Link_Wheel_Left/LConn1 -- Joint_Wheel_Left1/RConn1
  Simulink-PS Converter6/RConn1 -- Joint14/LConn2
  Link5/LConn1 -- Joint12/RConn1
  Joint13/RConn3 -- PS-Simulink Converter12/LConn1
  Link7/RConn1 -- Joint7_End-box/LConn1
  world-mobile-Transform/RConn2 -- PS-Simulink Converter30/LConn1
  PS-Simulink Converter14/LConn1 -- Joint12/RConn3
  Link_Wheel_Right/RConn1 -- Spatial Contact Force/RConn1
  Link_Rear1/RConn1 -- Joint_Rear4/LConn1
  Link_Rear2/LConn1 -- Joint_Rear4/RConn1
  Simulink-PS Converter1/RConn1 -- Joint9/LConn2
  PS-Simulink Converter22/LConn1 -- Joint8/RConn3
  Solver Configuration1/RConn1 -- room/RConn1 -- ball/LConn1 -- World1/RConn1 -- MechanismConfiguration1/RConn1 -- world-end-Transform/LConn1 -- world-mobile-Transform/LConn1 -- world-base/LConn1
  world-mobile-Transform1/RConn2 -- PS-Simulink Converter38/LConn1
  Link1/LConn1 -- Joint8/RConn1
  Joint10/RConn2 -- PS-Simulink Converter4/LConn1
  Link_Rear2/RConn1 -- Spatial Contact Force2/RConn1
  Link6/RConn1 -- Joint14/LConn1
  Link2/LConn1 -- Joint9/RConn1
  PS-Simulink Converter37/LConn1 -- world-mobile-Transform1/RConn5
  world-end-Transform/RConn1 -- Joint7_End-box/RConn1 -- end-box/LConn1 -- world-mobile-Transform1/RConn1
  Link_Wheel_Left/RConn1 -- Spatial Contact Force1/RConn1
  Simulink-PS Converter/RConn1 -- Joint8/LConn2
  Simulink-PS Converter4/RConn1 -- Joint12/LConn2
  Joint9/RConn2 -- PS-Simulink Converter3/LConn1
  Joint_Wheel_Left1/RConn2 -- PS-Simulink Converter/LConn1
  Link6/LConn1 -- Joint13/RConn1
  Link3/LConn1 -- Joint10/RConn1
  world-mobile-Transform/RConn1 -- 6-DOF Joint/RConn1 -- Frame_Base/LConn1 -- world-mobile-Transform1/LConn1
  Joint12/RConn2 -- PS-Simulink Converter6/LConn1
  Spatial Contact Force/LConn1 -- Spatial Contact Force1/LConn1 -- Spatial Contact Force2/LConn1 -- room/LConn1
  PS-Simulink Converter5/LConn1 -- Joint11/RConn2
  world-end-Transform/RConn5 -- PS-Simulink Converter33/LConn1
  Joint9/RConn3 -- PS-Simulink Converter20/LConn1
  PS-Simulink Converter18/LConn1 -- Joint10/RConn3
  Link5/RConn1 -- Joint13/LConn1
  Joint_Wheel_Right1/RConn2 -- PS-Simulink Converter1/LConn1
  Link4/RConn1 -- Joint12/LConn1
  Link1/RConn1 -- Joint9/LConn1
  Link_Wheel_Right/LConn1 -- Joint_Wheel_Right1/RConn1
  Link2/RConn1 -- Joint10/LConn1
  PS-Simulink Converter36/LConn1 -- world-mobile-Transform1/RConn4
  Link7/LConn1 -- Joint14/RConn1
  Simulink-PS Converter3/RConn1 -- Joint11/LConn2
  Simulink-PS Converter8/RConn1 -- Joint_Wheel_Right1/LConn2
  PS-Simulink Converter35/LConn1 -- world-mobile-Transform1/RConn3
  Joint14/RConn3 -- PS-Simulink Converter9/LConn1
  Joint_Wheel_Left1/LConn2 -- Simulink-PS Converter7/RConn1
  Joint10/LConn2 -- Simulink-PS Converter2/RConn1
  PS-Simulink Converter23/LConn1 -- Joint_Wheel_Left1/RConn3
  Joint8/RConn2 -- PS-Simulink Converter2/LConn1
  PS-Simulink Converter25/LConn1 -- Joint_Wheel_Right1/RConn3
  Joint11/RConn3 -- PS-Simulink Converter16/LConn1
  Frame_Base/LConn4 -- Joint_Rear3/LConn1
  Link3/RConn1 -- Joint11/LConn1
  Frame_Base/LConn3 -- Joint_Wheel_Left1/LConn1
  Frame_Base/RConn1 -- Joint8/LConn1
  world-mobile-Transform/RConn6 -- PS-Simulink Converter27/LConn1
  world-mobile-Transform/RConn8 -- PS-Simulink Converter29/LConn1
  world-mobile-Transform/RConn7 -- PS-Simulink Converter28/LConn1
  world-mobile-Transform/RConn4 -- PS-Simulink Converter11/LConn1
  world-mobile-Transform/RConn5 -- PS-Simulink Converter13/LConn1
  world-mobile-Transform/RConn3 -- PS-Simulink Converter10/LConn1
  world-mobile-Transform/RConn10 -- PS-Simulink Converter17/LConn1
  world-mobile-Transform/RConn11 -- PS-Simulink Converter19/LConn1
  world-mobile-Transform/RConn9 -- PS-Simulink Converter15/LConn1
  world-end-Transform/RConn7 -- PS-Simulink Converter24/LConn1
  world-end-Transform/RConn8 -- PS-Simulink Converter26/LConn1
  world-end-Transform/RConn6 -- PS-Simulink Converter21/LConn1
  world-end-Transform/RConn9 -- PS-Simulink Converter39/LConn1
  world-end-Transform/RConn10 -- PS-Simulink Converter40/LConn1
  world-end-Transform/RConn11 -- PS-Simulink Converter41/LConn1
  world-mobile-Transform1/RConn6 -- PS-Simulink Converter42/LConn1
  world-mobile-Transform1/RConn7 -- PS-Simulink Converter43/LConn1
  world-mobile-Transform1/RConn8 -- PS-Simulink Converter44/LConn1
  world-mobile-Transform1/RConn10 -- PS-Simulink Converter46/LConn1
  world-mobile-Transform1/RConn11 -- PS-Simulink Converter47/LConn1
  world-mobile-Transform1/RConn9 -- PS-Simulink Converter45/LConn1
  6-DOF Joint/LConn1 -- world-base/RConn1

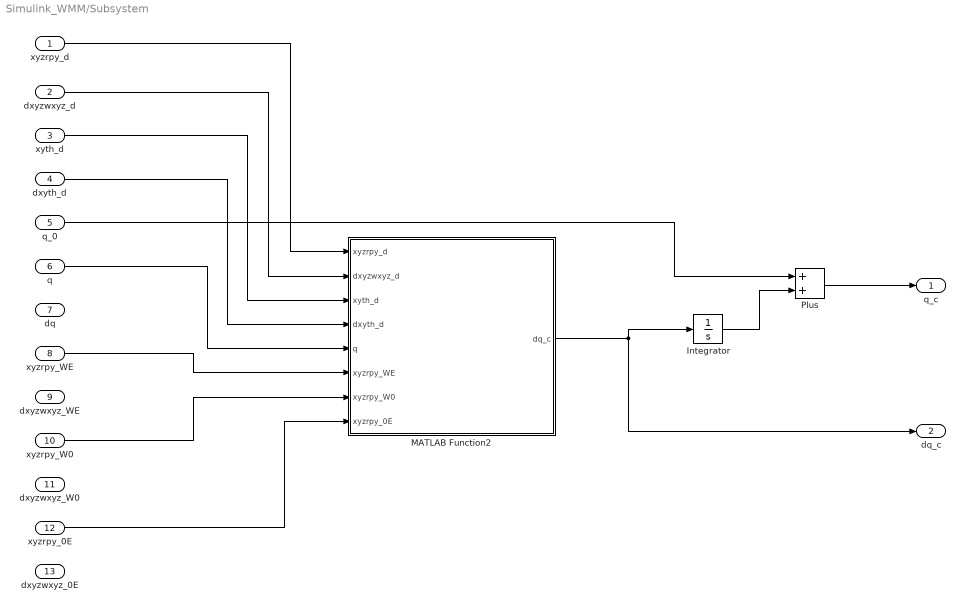
== system Simulink_WMM/Subsystem ==
  xyzrpy_d : Inport
  dxyzwxyz_d : Inport  Port=2
  xyth_d : Inport  Port=3
  dxyth_d : Inport  Port=4
  q_0 : Inport  Port=5
  q : Inport  Port=6
  dq : Inport  Port=7
  xyzrpy_WE : Inport  Port=8
  dxyzwxyz_WE : Inport  Port=9
  xyzrpy_W0 : Inport  Port=10
  dxyzwxyz_W0 : Inport  Port=11
  xyzrpy_0E : Inport  Port=12
  dxyzwxyz_0E : Inport  Port=13
  Integrator : Integrator
  MATLAB Function2 : MATLAB Function  TreatAsAtomicUnit=on
  Plus : Sum
  q_c : Outport
  dq_c : Outport  Port=2
  wires:
  xyzrpy_d/1 -> MATLAB Function2/1(xyzrpy_d)
  dxyzwxyz_d/1 -> MATLAB Function2/2(dxyzwxyz_d)
  xyzrpy_WE/1 -> MATLAB Function2/6(xyzrpy_WE)
  q/1 -> MATLAB Function2/5(q)
  xyzrpy_W0/1 -> MATLAB Function2/7(xyzrpy_W0)
  MATLAB Function2/1(dq_c) -> Integrator/1, dq_c/1
  Integrator/1 -> Plus/2
  Plus/1 -> q_c/1
  q_0/1 -> Plus/1
  xyth_d/1 -> MATLAB Function2/3(xyth_d)
  dxyth_d/1 -> MATLAB Function2/4(dxyth_d)
  xyzrpy_0E/1 -> MATLAB Function2/8(xyzrpy_0E)

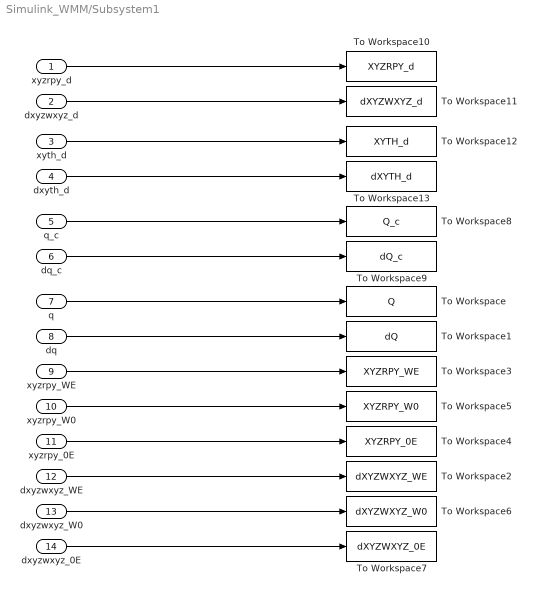
== system Simulink_WMM/Subsystem1 ==
  xyzrpy_d : Inport
  dxyzwxyz_d : Inport  Port=2
  xyth_d : Inport  Port=3
  dxyth_d : Inport  Port=4
  q_c : Inport  Port=5
  dq_c : Inport  Port=6
  q : Inport  Port=7
  dq : Inport  Port=8
  xyzrpy_WE : Inport  Port=9
  xyzrpy_W0 : Inport  Port=10
  xyzrpy_0E : Inport  Port=11
  dxyzwxyz_WE : Inport  Port=12
  dxyzwxyz_W0 : Inport  Port=13
  dxyzwxyz_0E : Inport  Port=14
  To Workspace : ToWorkspace  VariableName=Q  SaveFormat=Timeseries  SampleTime=-1
  To Workspace1 : ToWorkspace  VariableName=dQ  SaveFormat=Timeseries  SampleTime=-1
  To Workspace10 : ToWorkspace  VariableName=XYZRPY_d  SaveFormat=Timeseries  SampleTime=-1
  To Workspace11 : ToWorkspace  VariableName=dXYZWXYZ_d  SaveFormat=Timeseries  SampleTime=-1
  To Workspace12 : ToWorkspace  VariableName=XYTH_d  SaveFormat=Timeseries  SampleTime=-1
  To Workspace13 : ToWorkspace  VariableName=dXYTH_d  SaveFormat=Timeseries  SampleTime=-1
  To Workspace2 : ToWorkspace  VariableName=dXYZWXYZ_WE  SaveFormat=Timeseries  SampleTime=-1
  To Workspace3 : ToWorkspace  VariableName=XYZRPY_WE  SaveFormat=Timeseries  SampleTime=-1
  To Workspace4 : ToWorkspace  VariableName=XYZRPY_0E  SaveFormat=Timeseries  SampleTime=-1
  To Workspace5 : ToWorkspace  VariableName=XYZRPY_W0  SaveFormat=Timeseries  SampleTime=-1
  To Workspace6 : ToWorkspace  VariableName=dXYZWXYZ_W0  SaveFormat=Timeseries  SampleTime=-1
  To Workspace7 : ToWorkspace  VariableName=dXYZWXYZ_0E  SaveFormat=Timeseries  SampleTime=-1
  To Workspace8 : ToWorkspace  VariableName=Q_c  SaveFormat=Timeseries  SampleTime=-1
  To Workspace9 : ToWorkspace  VariableName=dQ_c  SaveFormat=Timeseries  SampleTime=-1
  wires:
  q/1 -> To Workspace/1
  dxyzwxyz_WE/1 -> To Workspace2/1
  xyzrpy_WE/1 -> To Workspace3/1
  xyzrpy_0E/1 -> To Workspace4/1
  dxyzwxyz_W0/1 -> To Workspace6/1
  xyzrpy_W0/1 -> To Workspace5/1
  dxyzwxyz_0E/1 -> To Workspace7/1
  dq/1 -> To Workspace1/1
  dq_c/1 -> To Workspace9/1
  q_c/1 -> To Workspace8/1
  dxyzwxyz_d/1 -> To Workspace11/1
  xyzrpy_d/1 -> To Workspace10/1
  dxyth_d/1 -> To Workspace13/1
  xyth_d/1 -> To Workspace12/1

== system Simulink_WMM/Subsystem3 ==
  MATLAB Function : MATLAB Function  TreatAsAtomicUnit=on
  clock : Clock
      settings: Decimation=100
  xyzrpy_d : Outport
  dxyzwxyz_d : Outport  Port=2
  xyth_d : Outport  Port=3
  dxyth_d : Outport  Port=4
  q_0 : Outport  Port=5
  wires:
  clock/1 -> MATLAB Function/1(t)
  MATLAB Function/1(xyzrpy_d) -> xyzrpy_d/1
  MATLAB Function/3(xyth_d) -> xyth_d/1
  MATLAB Function/2(dxyzwxyz_d) -> dxyzwxyz_d/1
  MATLAB Function/4(dxyth_d) -> dxyth_d/1
  MATLAB Function/5(q_0) -> q_0/1
